simulink model "TPGCI_STM32_4"  (R2024a)
settings: Solver=FixedStepDiscrete  StartTime=0.0  StopTime=10.0  FixedStep=100e-6  RelTol=1e-3
undefined symbols (not defined in the file): DiscIntNeverNeededParam
libraries: slpidlib x3, spsabctodq0Lib x2, spsdq0toabcLib x1
settings Model: Creator=mahes  LastModifiedBy=mahes
settings OptimizationCC: DefaultParameterBehavior=Inlined  UseDivisionForNetSlopeComputation=on  GainParamInheritBuiltInType=on  UseFloatMulNetSlope=on  UseSpecifiedMinMax=on  InlineInvariantSignals=on  PassReuseOutputArgsAs=Individual arguments  ZeroExternalMemoryAtStartup=off  ZeroInternalMemoryAtStartup=off  NoFixptDivByZeroProtection=on  EfficientFloat2IntCast=on  LifeSpan=1  OptimizeBlockOrder=speed  DifferentSizesBufferReuse=on  EfficientTunableParamExpr=on
settings DebuggingCC: ParameterTunabilityLossMsg=error
settings HardwareCC: ProdBitPerPointer=32  ProdBitPerSizeT=32  ProdBitPerPtrDiffT=32  ProdLargestAtomicInteger=Long  ProdLargestAtomicFloat=Double  ProdWordSize=32  ProdLongLongMode=on  ProdHWDeviceType=ARM Compatible->ARM Cortex-M
settings SFSimCC: MATLABDynamicMemAlloc=off
settings RTWCC: Description=Embedded Coder  SystemTargetFile=ert.tlc  TemplateMakefile=ert_default_tmf  GenerateReport=on  BuildConfiguration=Faster Runs  LaunchReport=on  DataTypeReplacement=CDataTypesFixedWidth  CheckMdlBeforeBuild=Warning
settings CodeAppCC: ForceParamTrailComments=on  IgnoreCustomStorageClasses=off  OperatorAnnotations=on  SimulinkDataObjDesc=on  SFDataObjDesc=on  CustomSymbolStrGlobalVar=rt$N$M  CustomSymbolStrType=$N$M  CustomSymbolStrFcn=$N$M$F  CustomSymbolStrMacro=$N$M  InsertBlockDesc=on
settings ERTTargetCC: TargetLangStandard=C99 (ISO)  GenerateSampleERTMain=on  IncludeMdlTerminateFcn=off  CombineSignalStateStructs=on  SuppressErrorStatus=on  SupportAbsoluteTime=off  SupportNonFinite=off  SupportComplex=off  InlinedParameterPlacement=NonHierarchical  ERTCustomFileTemplate=example_file_process.tlc  ERTFilePackagingFormat=CompactWithDataFile  MaxIdInt64=INT64_MAX  MinIdInt64=INT64_MIN  MaxIdUint64=UINT64_MAX  MaxIdInt32=INT32_MAX  MinIdInt32=INT32_MIN  MaxIdUint32=UINT32_MAX  MaxIdInt16=INT16_MAX  MinIdInt16=INT16_MIN  MaxIdUint16=UINT16_MAX  MaxIdInt8=INT8_MAX  MinIdInt8=INT8_MIN  MaxIdUint8=UINT8_MAX

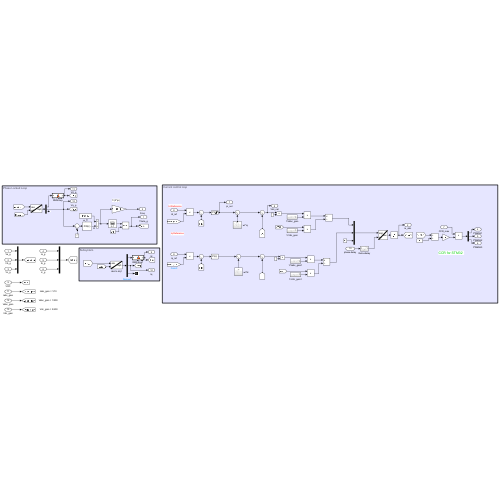
[thumbnail: Simulink's stored preview of the top-level diagram]
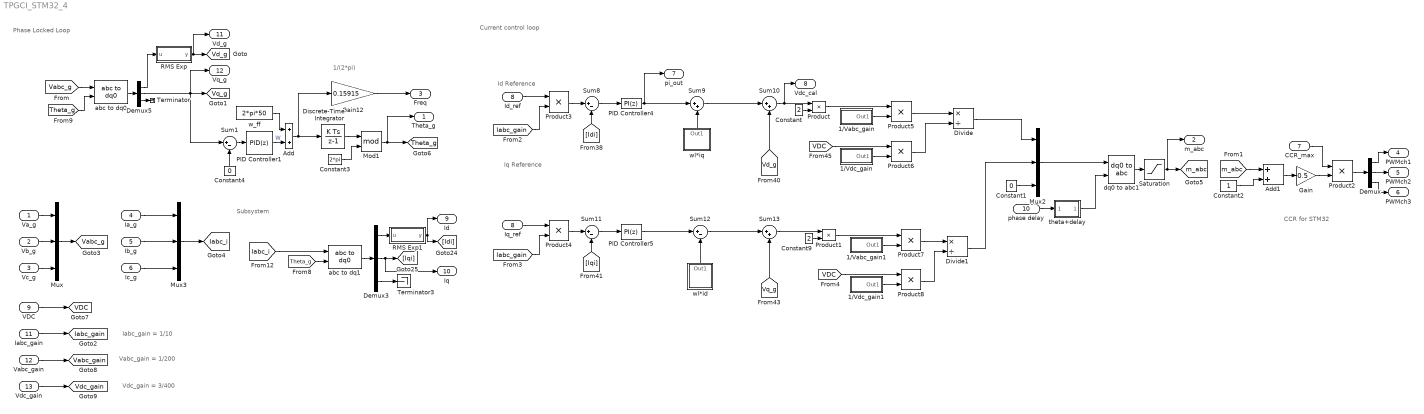
== system TPGCI_STM32_4 ==
  note: Vdc_gain = 3/400
  note: Vabc_gain = 1/200
  note: Iabc_gain = 1/10
  note: 1/(2*pi)
  note: Current control loop
  note: Subsystem
  note: CCR for STM32
  note: Iq Reference
  note: Id Reference
  note: Phase Locked Loop
  Va_g : Inport
  Vb_g : Inport  Port=2
  Vc_g : Inport  Port=3
  Ia_g : Inport  Port=4
  Ib_g : Inport  Port=5
  Ic_g : Inport  Port=6
  CCR_max : Inport  Port=7
  Id_ref : Inport  Port=8
  VDC : Inport  Port=9
  phase delay : Inport  Port=10
  Iabc_gain : Inport  Port=11
  Vabc_gain : Inport  Port=12
  Vdc_gain : Inport  Port=13
  1/Vabc_gain : Subsystem
  1/Vabc_gain1 : Subsystem
  1/Vdc_gain : Subsystem
  1/Vdc_gain1 : Subsystem
  Add : Sum
  Add1 : Sum
  Constant : Constant  Value=2
  Constant1 : Constant  Value=0
  Constant2 : Constant
  Constant3 : Constant  Value=2*pi
  Constant4 : Constant  Value=0
  Constant9 : Constant  Value=2
  Demux : Demux  Outputs=3
  Demux3 : Demux  Outputs=3
  Demux5 : Demux  Outputs=3
  Discrete-Time Integrator : DiscreteIntegrator  SampleTime=100e-6  ICPrevOutput=DiscIntNeverNeededParam  ICPrevScaledInput=DiscIntNeverNeededParam
  Divide : Product  Inputs=*/
  Divide1 : Product  Inputs=*/
  Gain : Gain  Gain=0.5
  Gain12 : Gain  Gain=0.15915
  Iq_ref : InportShadow  Port=8
  Mod1 : Math  Operator=mod
  Mux : Mux  Inputs=3
  Mux2 : Mux  Inputs=3
  Mux3 : Mux  Inputs=3
  PID Controller1 : slpidlib/PID Controller  Controller=PID  Form=Parallel  TimeDomain=Discrete-time  UseExternalTs=off  SampleTime=100e-6  IntegratorMethod=Forward Euler  FilterMethod=Forward Euler  ControllerParametersSource=internal  P=10  I=10000  UseKiTs=off  D=0  UseExternalDerivativeSource=off  N=100  UseFilter=on  TunerSelectOption=Transfer Function Based (PID Tuner App)  InitialConditionSource=internal  InitialConditionForIntegrator=0  InitialConditionForFilter=0  DifferentiatorICPrevScaledInput=0  ExternalReset=none  TrackingMode=off  Kt=1  LimitOutput=off  SatLimitsSource=internal  UpperSaturationLimit=inf  LowerSaturationLimit=-inf  LinearizeAsGain=on  AntiWindupMode=none  Kb=1  LimitIntegrator=off  UpperIntegratorSaturationLimit=inf  LowerIntegratorSaturationLimit=-inf  POutMin=[]  POutMax=[]  IOutMin=[]  IOutMax=[]  DOutMin=[]  DOutMax=[]  NOutMin=[]  NOutMax=[]  SumOutMin=[]  SumOutMax=[]  SaturationOutMin=[]  SaturationOutMax=[]  PParamMin=[]  PParamMax=[]  IParamMin=[]  IParamMax=[]  DParamMin=[]  DParamMax=[]  NParamMin=[]  NParamMax=[]  KbParamMin=[]  KbParamMax=[]  KtParamMin=[]  KtParamMax=[]  KbOutMin=[]  KbOutMax=[]  KtOutMin=[]  KtOutMax=[]  IntegratorOutMin=[]  IntegratorOutMax=[]  FilterOutMin=[]  FilterOutMax=[]  SumI1OutMin=[]  SumI1OutMax=[]  SumI2OutMin=[]  SumI2OutMax=[]  SumI3OutMin=[]  SumI3OutMax=[]  SumI4OutMin=[]  SumI4OutMax=[]  SumDOutMin=[]  SumDOutMax=[]  DifferentiatorOutMin=[]  DifferentiatorOutMax=[]  FilterDiffOutCoefMin=[]  FilterDiffOutCoefMax=[]  ReciprocalOutMin=[]  ReciprocalOutMax=[]  SumDenOutMin=[]  SumDenOutMax=[]  SumNumOutMin=[]  SumNumOutMax=[]  DivideOutMin=[]  DivideOutMax=[]  UdiffTsProdOutMin=[]  UdiffTsProdOutMax=[]  NTsProdOutMin=[]  NTsProdOutMax=[]  UintegralTsProdOutMin=[]  UintegralTsProdOutMax=[]  UngainTsProdOutMin=[]  UngainTsProdOutMax=[]  ClampingZeroOutDataTypeStr=Inherit: Inherit via back propagation  ClampingZeroOutMin=[]  ClampingZeroOutMax=[]  FilterDenConstantOutDataTypeStr=Inherit: Inherit via back propagation  FilterDenConstantOutMin=[]  FilterDenConstantOutMax=[]  PCopyOutDataTypeStr=Inherit: Inherit via back propagation  PCopyOutMin=[]  PCopyOutMax=[]  NCopyOutDataTypeStr=Inherit: Inherit via back propagation  NCopyOutMin=[]  NCopyOutMax=[]  IntegratorContinuousStateAttributes=''  IntegratorStateMustResolveToSignalObject=off  IntegratorRTWStateStorageClass=Auto  FilterContinuousStateAttributes=''  FilterStateMustResolveToSignalObject=off  FilterRTWStateStorageClass=Auto  ParallelPVariant=InternalParameters  IdealPVariant=Disabled  IVariant=InternalParameters  DVariant=InternalParameters  IntegratorVariant=Discrete  SatVariant=Disabled  AWVariant=Passthrough  PCopyVariant=Disabled  TRVariant=Disabled  FdbkBlocksVariant=Forward  IdealPFdbkVariant=Disabled  SatFdbkVariant=Disabled  DerivativeFilterVariant=ForwardEulerFilter  NVariant=InternalParameters  NCopyVariant=Disabled  FilterICVariant=InternalICsFilter  IntegratorICVariant=InternalICs  ExternalResetVariant=Disabled  TRSumVariant=Passthrough  SumFdbkVariant=Disabled  SumVariant=Sum_PID  TsampFilterVariant=InternalTs  TsampNgainVariant=Passthrough  TsampIntegralVariant=Disabled_SignalSpec  ExternalSaturationOutDataTypeStr=Inherit: Same as second input  DerivativeSourceVariant=ErrorSignal
  PID Controller4 : slpidlib/PID Controller  Controller=PI  Form=Parallel  TimeDomain=Discrete-time  UseExternalTs=off  SampleTime=100e-6  IntegratorMethod=Forward Euler  FilterMethod=Forward Euler  ControllerParametersSource=internal  P=1  I=100  UseKiTs=off  D=0  UseExternalDerivativeSource=off  N=100  UseFilter=on  TunerSelectOption=Transfer Function Based (PID Tuner App)  InitialConditionSource=internal  InitialConditionForIntegrator=0  InitialConditionForFilter=0  DifferentiatorICPrevScaledInput=0  ExternalReset=none  TrackingMode=off  Kt=1  LimitOutput=on  SatLimitsSource=internal  UpperSaturationLimit=10  LowerSaturationLimit=-10  LinearizeAsGain=on  AntiWindupMode=none  Kb=1  LimitIntegrator=on  UpperIntegratorSaturationLimit=10  LowerIntegratorSaturationLimit=-10  POutMin=[]  POutMax=[]  IOutMin=[]  IOutMax=[]  DOutMin=[]  DOutMax=[]  NOutMin=[]  NOutMax=[]  SumOutMin=[]  SumOutMax=[]  SaturationOutMin=[]  SaturationOutMax=[]  PParamMin=[]  PParamMax=[]  IParamMin=[]  IParamMax=[]  DParamMin=[]  DParamMax=[]  NParamMin=[]  NParamMax=[]  KbParamMin=[]  KbParamMax=[]  KtParamMin=[]  KtParamMax=[]  KbOutMin=[]  KbOutMax=[]  KtOutMin=[]  KtOutMax=[]  IntegratorOutMin=[]  IntegratorOutMax=[]  FilterOutMin=[]  FilterOutMax=[]  SumI1OutMin=[]  SumI1OutMax=[]  SumI2OutMin=[]  SumI2OutMax=[]  SumI3OutMin=[]  SumI3OutMax=[]  SumI4OutMin=[]  SumI4OutMax=[]  SumDOutMin=[]  SumDOutMax=[]  DifferentiatorOutMin=[]  DifferentiatorOutMax=[]  FilterDiffOutCoefMin=[]  FilterDiffOutCoefMax=[]  ReciprocalOutMin=[]  ReciprocalOutMax=[]  SumDenOutMin=[]  SumDenOutMax=[]  SumNumOutMin=[]  SumNumOutMax=[]  DivideOutMin=[]  DivideOutMax=[]  UdiffTsProdOutMin=[]  UdiffTsProdOutMax=[]  NTsProdOutMin=[]  NTsProdOutMax=[]  UintegralTsProdOutMin=[]  UintegralTsProdOutMax=[]  UngainTsProdOutMin=[]  UngainTsProdOutMax=[]  ClampingZeroOutDataTypeStr=Inherit: Inherit via back propagation  ClampingZeroOutMin=[]  ClampingZeroOutMax=[]  FilterDenConstantOutDataTypeStr=Inherit: Inherit via back propagation  FilterDenConstantOutMin=[]  FilterDenConstantOutMax=[]  PCopyOutDataTypeStr=Inherit: Inherit via back propagation  PCopyOutMin=[]  PCopyOutMax=[]  NCopyOutDataTypeStr=Inherit: Inherit via back propagation  NCopyOutMin=[]  NCopyOutMax=[]  IntegratorContinuousStateAttributes=''  IntegratorStateMustResolveToSignalObject=off  IntegratorRTWStateStorageClass=Auto  FilterContinuousStateAttributes=''  FilterStateMustResolveToSignalObject=off  FilterRTWStateStorageClass=Auto  ParallelPVariant=InternalParameters  IdealPVariant=Disabled  IVariant=InternalParameters  DVariant=Disabled  IntegratorVariant=Discrete  SatVariant=Enabled  AWVariant=Passthrough  PCopyVariant=Disabled  TRVariant=Disabled  FdbkBlocksVariant=Forward  IdealPFdbkVariant=Disabled  SatFdbkVariant=Disabled  DerivativeFilterVariant=Disabled  NVariant=Disabled  NCopyVariant=Disabled_SignalSpec  FilterICVariant=Disabled  IntegratorICVariant=InternalICs  ExternalResetVariant=Disabled  TRSumVariant=Passthrough  SumFdbkVariant=Disabled  SumVariant=Sum_PI  TsampFilterVariant=InternalTs  TsampNgainVariant=Passthrough  TsampIntegralVariant=Disabled_SignalSpec  ExternalSaturationOutDataTypeStr=Inherit: Same as second input  DerivativeSourceVariant=Disabled
  PID Controller5 : slpidlib/PID Controller  Controller=PI  Form=Parallel  TimeDomain=Discrete-time  UseExternalTs=off  SampleTime=100e-6  IntegratorMethod=Forward Euler  FilterMethod=Forward Euler  ControllerParametersSource=internal  P=1  I=100  UseKiTs=off  D=0  UseExternalDerivativeSource=off  N=100  UseFilter=on  TunerSelectOption=Transfer Function Based (PID Tuner App)  InitialConditionSource=internal  InitialConditionForIntegrator=0  InitialConditionForFilter=0  DifferentiatorICPrevScaledInput=0  ExternalReset=none  TrackingMode=off  Kt=1  LimitOutput=off  SatLimitsSource=internal  UpperSaturationLimit=inf  LowerSaturationLimit=-inf  LinearizeAsGain=on  AntiWindupMode=none  Kb=1  LimitIntegrator=off  UpperIntegratorSaturationLimit=inf  LowerIntegratorSaturationLimit=-inf  POutMin=[]  POutMax=[]  IOutMin=[]  IOutMax=[]  DOutMin=[]  DOutMax=[]  NOutMin=[]  NOutMax=[]  SumOutMin=[]  SumOutMax=[]  SaturationOutMin=[]  SaturationOutMax=[]  PParamMin=[]  PParamMax=[]  IParamMin=[]  IParamMax=[]  DParamMin=[]  DParamMax=[]  NParamMin=[]  NParamMax=[]  KbParamMin=[]  KbParamMax=[]  KtParamMin=[]  KtParamMax=[]  KbOutMin=[]  KbOutMax=[]  KtOutMin=[]  KtOutMax=[]  IntegratorOutMin=[]  IntegratorOutMax=[]  FilterOutMin=[]  FilterOutMax=[]  SumI1OutMin=[]  SumI1OutMax=[]  SumI2OutMin=[]  SumI2OutMax=[]  SumI3OutMin=[]  SumI3OutMax=[]  SumI4OutMin=[]  SumI4OutMax=[]  SumDOutMin=[]  SumDOutMax=[]  DifferentiatorOutMin=[]  DifferentiatorOutMax=[]  FilterDiffOutCoefMin=[]  FilterDiffOutCoefMax=[]  ReciprocalOutMin=[]  ReciprocalOutMax=[]  SumDenOutMin=[]  SumDenOutMax=[]  SumNumOutMin=[]  SumNumOutMax=[]  DivideOutMin=[]  DivideOutMax=[]  UdiffTsProdOutMin=[]  UdiffTsProdOutMax=[]  NTsProdOutMin=[]  NTsProdOutMax=[]  UintegralTsProdOutMin=[]  UintegralTsProdOutMax=[]  UngainTsProdOutMin=[]  UngainTsProdOutMax=[]  ClampingZeroOutDataTypeStr=Inherit: Inherit via back propagation  ClampingZeroOutMin=[]  ClampingZeroOutMax=[]  FilterDenConstantOutDataTypeStr=Inherit: Inherit via back propagation  FilterDenConstantOutMin=[]  FilterDenConstantOutMax=[]  PCopyOutDataTypeStr=Inherit: Inherit via back propagation  PCopyOutMin=[]  PCopyOutMax=[]  NCopyOutDataTypeStr=Inherit: Inherit via back propagation  NCopyOutMin=[]  NCopyOutMax=[]  IntegratorContinuousStateAttributes=''  IntegratorStateMustResolveToSignalObject=off  IntegratorRTWStateStorageClass=Auto  FilterContinuousStateAttributes=''  FilterStateMustResolveToSignalObject=off  FilterRTWStateStorageClass=Auto  ParallelPVariant=InternalParameters  IdealPVariant=Disabled  IVariant=InternalParameters  DVariant=Disabled  IntegratorVariant=Discrete  SatVariant=Disabled  AWVariant=Passthrough  PCopyVariant=Disabled  TRVariant=Disabled  FdbkBlocksVariant=Forward  IdealPFdbkVariant=Disabled  SatFdbkVariant=Disabled  DerivativeFilterVariant=Disabled  NVariant=Disabled  NCopyVariant=Disabled_SignalSpec  FilterICVariant=Disabled  IntegratorICVariant=InternalICs  ExternalResetVariant=Disabled  TRSumVariant=Passthrough  SumFdbkVariant=Disabled  SumVariant=Sum_PI  TsampFilterVariant=InternalTs  TsampNgainVariant=Passthrough  TsampIntegralVariant=Disabled_SignalSpec  ExternalSaturationOutDataTypeStr=Inherit: Same as second input  DerivativeSourceVariant=Disabled
  Product{,1..8} (9 alike) : Product
  RMS Exp : MATLAB Function  TreatAsAtomicUnit=on
  RMS Exp1 : MATLAB Function  TreatAsAtomicUnit=on
  Saturation : Saturate  UpperLimit=0.95  LowerLimit=-0.95
  Sum{1,8,11..12} (4 alike) : Sum  Inputs=|+-
  Sum10 : Sum  Inputs=|++
  Sum13 : Sum  Inputs=|++
  Sum9 : Sum  Inputs=|++
  Terminator : Terminator
  Terminator3 : Terminator
  abc to dq0 : spsabctodq0Lib/abc to dq0  Alignment=90 degrees behind phase A axis
  abc to dq1 : spsabctodq0Lib/abc to dq0  Alignment=90 degrees behind phase A axis
  dq0 to abc1 : spsdq0toabcLib/dq0 to abc  Alignment=90 degrees behind phase A axis
  theta+delay : Subsystem
  w_ff : Constant  Value=2*pi*50
  wl*id : Subsystem
  wl*iq : Subsystem
  Theta_g : Outport
  m_abc : Outport  Port=2
  Freq : Outport  Port=3
  PWMch1 : Outport  Port=4
  PWMch2 : Outport  Port=5
  PWMch3 : Outport  Port=6
  pi_out : Outport  Port=7
  Vdc_cal : Outport  Port=8
  Id : Outport  Port=9
  Iq : Outport  Port=10
  Vd_g : Outport  Port=11
  Vq_g : Outport  Port=12
  tag scope: Iabc_gain=global, Iabc_i=global, Theta_g=global, VDC=global, Vabc_g=global, Vabc_gain=global, Vd_g=global, Vdc_gain=global, Vq_g=global, m_abc=global
  wires:
  [Iabc_i] -> abc to dq1/1
  Gain12/1 -> Freq/1
  Gain/1 -> Product2/2
  Constant2/1 -> Add1/2
  Divide1/1 -> Mux2/2
  Constant4/1 -> Sum1/2
  Product2/1 -> Demux/1
  CCR_max/1 -> Product2/1
  [m_abc] -> Add1/1
  Demux/2 -> PWMch2/1
  abc to dq1/1 -> Demux3/1
  [Vabc_g] -> abc to dq0/1
  Demux/1 -> PWMch1/1
  Vb_g/1 -> Mux/2
  Sum11/1 -> PID Controller5/1
  Constant/1 -> Product/2
  Sum9/1 -> Sum10/1
  w_ff/1 -> Add/1
  VDC/1 -> [VDC]
  Sum10/1 -> Product/1, Vdc_cal/1
  Sum13/1 -> Product1/1
  Mux3/1 -> [Iabc_i]
  dq0 to abc1/1 -> Saturation/1
  [Theta_g] -> abc to dq0/2
  Ib_g/1 -> Mux3/2
  PID Controller4/1 -> pi_out/1, Sum9/1
  Constant3/1 -> Mod1/2
  Demux3/3 -> Terminator3/1
  Add1/1 -> Gain/1
  Sum1/1 -> PID Controller1/1
  Va_g/1 -> Mux/1
  [Theta_g] -> abc to dq1/2
  PID Controller1/1 -> Add/2  "W"
  Demux3/2 -> Iq/1, [Iqi]
  Ic_g/1 -> Mux3/3
  Discrete-Time Integrator/1 -> Mod1/1
  abc to dq0/1 -> Demux5/1
  Divide/1 -> Mux2/1
  Demux5/2 -> Sum1/1, Vq_g/1, [Vq_g]
  [Iqi] -> Sum11/2
  [Vq_g] -> Sum13/2
  [Idi] -> Sum8/2
  Mod1/1 -> [Theta_g], Theta_g/1
  Mux2/1 -> dq0 to abc1/1
  PID Controller5/1 -> Sum12/1
  Saturation/1 -> m_abc/1, [m_abc]
  Mux/1 -> [Vabc_g]
  Sum8/1 -> PID Controller4/1
  Constant9/1 -> Product1/2
  Sum12/1 -> Sum13/1
  Vc_g/1 -> Mux/3
  [Vd_g] -> Sum10/2
  Demux/3 -> PWMch3/1
  Ia_g/1 -> Mux3/1
  Add/1 -> Gain12/1, Discrete-Time Integrator/1
  Constant1/1 -> Mux2/3
  Demux5/3 -> Terminator/1
  Demux5/1 -> RMS Exp/1(u)
  RMS Exp/1(y) -> Vd_g/1, [Vd_g]
  Id_ref/1 -> Product3/1
  Iabc_gain/1 -> [Iabc_gain]
  Vabc_gain/1 -> [Vabc_gain]
  Vdc_gain/1 -> [Vdc_gain]
  [Iabc_gain] -> Product3/2
  Product3/1 -> Sum8/1
  Iq_ref/1 -> Product4/1
  [Iabc_gain] -> Product4/2
  Product4/1 -> Sum11/1
  Product5/1 -> Divide/1
  Product/1 -> Product5/1
  wl*iq/1(Out1) -> Sum9/2
  wl*id/1(Out1) -> Sum12/2
  1/Vabc_gain/1(Out1) -> Product5/2
  [VDC] -> Product6/1
  1/Vdc_gain/1(Out1) -> Product6/2
  Product6/1 -> Divide/2
  [VDC] -> Product8/1
  Product1/1 -> Product7/1
  1/Vabc_gain1/1(Out1) -> Product7/2
  Product7/1 -> Divide1/1
  1/Vdc_gain1/1(Out1) -> Product8/2
  Product8/1 -> Divide1/2
  theta+delay/1(Out1) -> dq0 to abc1/2
  phase delay/1 -> theta+delay/1(Inport)
  Demux3/1 -> RMS Exp1/1(u)
  RMS Exp1/1(y) -> Id/1, [Idi]

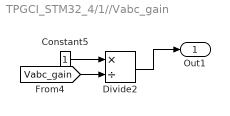
== system TPGCI_STM32_4/1//Vabc_gain ==
  Constant5 : Constant
  Divide2 : Product  Inputs=*/
  Out1 : Outport
  wires:
  Divide2/1 -> Out1/1
  [Vabc_gain] -> Divide2/2
  Constant5/1 -> Divide2/1

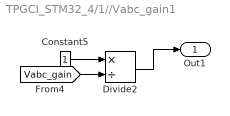
== system TPGCI_STM32_4/1//Vabc_gain1 ==
  Constant5 : Constant
  Divide2 : Product  Inputs=*/
  Out1 : Outport
  wires:
  Divide2/1 -> Out1/1
  [Vabc_gain] -> Divide2/2
  Constant5/1 -> Divide2/1

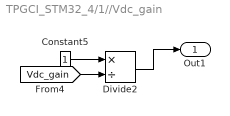
== system TPGCI_STM32_4/1//Vdc_gain ==
  Constant5 : Constant
  Divide2 : Product  Inputs=*/
  Out1 : Outport
  wires:
  Constant5/1 -> Divide2/1
  [Vdc_gain] -> Divide2/2
  Divide2/1 -> Out1/1

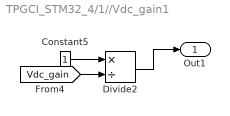
== system TPGCI_STM32_4/1//Vdc_gain1 ==
  Constant5 : Constant
  Divide2 : Product  Inputs=*/
  Out1 : Outport
  wires:
  Constant5/1 -> Divide2/1
  [Vdc_gain] -> Divide2/2
  Divide2/1 -> Out1/1

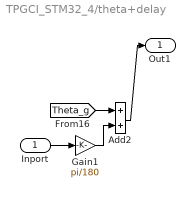
== system TPGCI_STM32_4/theta+delay ==
  Inport : Inport
  Add2 : Sum
  Gain1 : Gain  Gain=pi/180
  Out1 : Outport
  wires:
  Gain1/1 -> Add2/2
  Inport/1 -> Gain1/1
  Add2/1 -> Out1/1
  [Theta_g] -> Add2/1

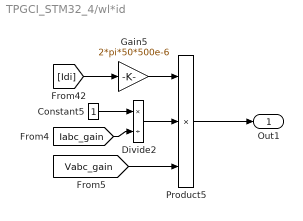
== system TPGCI_STM32_4/wl*id ==
  Constant5 : Constant
  Divide2 : Product  Inputs=*/
  Gain5 : Gain  Gain=2*pi*50*500e-6
  Product5 : Product  Inputs=3
  Out1 : Outport
  wires:
  Divide2/1 -> Product5/2
  [Iabc_gain] -> Divide2/2
  [Vabc_gain] -> Product5/3
  [Idi] -> Gain5/1
  Constant5/1 -> Divide2/1
  Product5/1 -> Out1/1
  Gain5/1 -> Product5/1

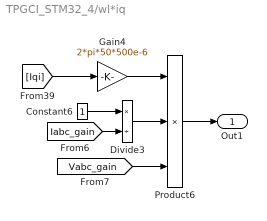
== system TPGCI_STM32_4/wl*iq ==
  Constant6 : Constant
  Divide3 : Product  Inputs=*/
  Gain4 : Gain  Gain=2*pi*50*500e-6
  Product6 : Product  Inputs=3
  Out1 : Outport
  wires:
  Divide3/1 -> Product6/2
  [Iabc_gain] -> Divide3/2
  [Iqi] -> Gain4/1
  Constant6/1 -> Divide3/1
  Gain4/1 -> Product6/1
  [Vabc_gain] -> Product6/3
  Product6/1 -> Out1/1

== matlab function TPGCI_STM32_4/RMS Exp ==
  settings: updateMethod=DISCRETE
  data: y output; u input
function y = movingRMSExp(u)
    % y = movingRMSExp(u, alpha)
    % This function computes the exponential moving RMS of the input signal `u`.
    % The parameter `alpha` is the smoothing factor (0 < alpha <= 1).
    % A higher `alpha` gives more weight to recent values.

    % Persistent variables to maintain state between calls
    persistent rmsSquared

    % Initialize the exponential moving RMS on the first call
    if isempty(rmsSquared)
        rmsSquared = u^2; % Initialize with the square of the first value
    end

    % Update the exponentially weighted RMS squared
    rmsSquared = 0.01 * u^2 + (1 - 0.01) * rmsSquared;

    % Compute the RMS as the square root of the weighted sum
    y = sqrt(rmsSquared);
end

== matlab function TPGCI_STM32_4/RMS Exp1 ==
  settings: updateMethod=DISCRETE
  data: y output; u input
function y = movingRMSExp(u)
    % y = movingRMSExp(u, alpha)
    % This function computes the exponential moving RMS of the input signal `u`.
    % The parameter `alpha` is the smoothing factor (0 < alpha <= 1).
    % A higher `alpha` gives more weight to recent values.

    % Persistent variables to maintain state between calls
    persistent rmsSquared

    % Initialize the exponential moving RMS on the first call
    if isempty(rmsSquared)
        rmsSquared = u^2; % Initialize with the square of the first value
    end

    % Update the exponentially weighted RMS squared
    rmsSquared = 0.01 * u^2 + (1 - 0.01) * rmsSquared;

    % Compute the RMS as the square root of the weighted sum
    y = sqrt(rmsSquared);
end
